simulink model "Flipper"  (R2015a)
settings: Solver=ode45  StartTime=0.0  StopTime=10.0  RelTol=1e-3
libraries: vrlib x2
settings Model: Creator=john  LastModifiedBy=john

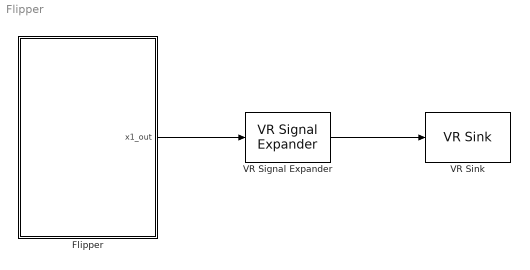
== system Flipper ==
  Flipper : Stateflow chart  TreatAsAtomicUnit=on
  VR Signal Expander : vrlib/VR Signal Expander  outwidth=3  outidx=[1 2]
  VR Sink : vrlib/VR Sink  InstantiateOnLoad=on  SampleTime=0.05  ViewEnable=on  RemoteChange=off  RemoteView=off  FieldsWritten=Ball.translation.3.1.1.double  WorldFileName=Table.wrl  AutoView=off  VideoDimensions=[]  AllowVariableSize=off
  wires:
  VR Signal Expander/1 -> VR Sink/1
  Flipper/1(x1_out) -> VR Signal Expander/1

== stateflow chart Flipper/Flipper ==
  settings: updateMethod=CONTINUOUS
  state Flipper
    during:
    x1_dot=v1;
    v1_dot=Acc();
    x1_out=x1;
  (default) -> Flipper : {Init();}
  Flipper -> Flipper [order 1] : [WandLKontakt()]
      | {WandLRefl()}
  Flipper -> Flipper [order 2] : [WandUKontakt()]
      | {WandURefl()}
  Flipper -> Flipper [order 3] : [WandRKontakt()]
      | {WandRRefl()}
  Flipper -> Flipper [order 4] : [HndKontakt()]
      | {HndRefl()}
  data: k function_output boolean; a function_output; k function_output boolean; k function_output boolean; k function_output boolean; R constant double =0.25; RHnd constant double =0.8; Hnd local double size=2,1; n1 local double size=2,1; n2 local double size=2,1; n3 local double size=2,1; p1 local double size=2,1; p2 local double size=2,1; p3 local double size=2,1; p4 local double size=2,1; t1 local double size=2,1; t2 local double size=2,1; t3 local double size=2,1; v1 local double size=2,1; x1 local double size=2,1; x1_out output double size=2,1
  data v1 settings: updateMethod=SF_CONTINUOUS_TIME_DATA
  data x1 settings: updateMethod=SF_CONTINUOUS_TIME_DATA
  function WandLRefl:
    | function WandLRefl
    | 
    | vt = v1' * t1;
    | vn = v1' * n1;
    | 
    | v1 = vt * t1 - vn * n1;
  function k = WandLKontakt:
    | function k = WandLKontakt
    | k = false;
    | if (abs((x1 - p1)' * n1) <= R && (v1' * n1) < 0)
    |     k = true;
    | end
  function Init:
    | function Init
    | 
    | x1 = [4; 5];
    | v1 = [0; 0];
    | 
    | p1 = [0; 5];
    | p2 = [5; 0];
    | p3 = [9; 0];
    | p4 = [10; 7];
    | Hnd = [6; 2.5];
    | 
    | t1 = (p2 - p1)/norm(p2 - p1);
    | n1 = [-t1(2); t1(1)];
    | 
    | t2 = (p3 - p2)/norm(p3 - p2);
    | n2 = [-t2(2); t2(1)];
    | 
    | t3 = (p4 - p3)/norm(p4 - p3);
    | n3 = [-t3(2); t3(1)];
  function a = Acc:
    | function a = Acc
    |  
    | a = [0; -1];
  function k = WandUKontakt:
    | function k = WandUKontakt
    | k = false;
    | if (abs((x1 - p2)' * n2) <= R && (v1' * n2) < 0)
    |     k = true; 
    | end
  function WandURefl:
    | function WandURefl
    | 
    | vt = v1' * t2;
    | vn = v1' * n2;
    | 
    | v1 = vt * t2 - vn * n2;
  function k = HndKontakt:
    | function k = HndKontakt
    | k = false;
    | 
    | n = (x1 - Hnd) / norm(x1 - Hnd);
    | t = [-n(2); n(1)];
    | 
    | if ( norm(Hnd - x1) <= RHnd + R && (v1' * n) < 0)
    |     k = true;
    | end
  function HndRefl:
    | function HndRefl
    | 
    | n = (Hnd - x1) / norm(Hnd - x1);
    | t = [n(2); -n(1)];
    | 
    | vt = v1' * t;
    | vn = v1' * n;
    | 
    | v1 = vt * t - vn * n;
  function k = WandRKontakt:
    | function k = WandRKontakt
    | k = false;
    | if (abs((x1 - p3)' * n3) <= R && (v1' * n3) < 0)
    |     k = true;
    | end
  function WandRRefl:
    | function WandRRefl
    | 
    | vt = v1' * t3;
    | vn = v1' * n3;
    | 
    | v1 = vt * t3 - vn * n3;
